simulink model "Dynamic_RLC_system"  (R2024a)
settings: Solver=VariableStepAuto  StartTime=0.0  StopTime=10.0  MaxStep=1e-3  RelTol=1e-3
settings Model: Creator=DELL  LastModifiedBy=DELL

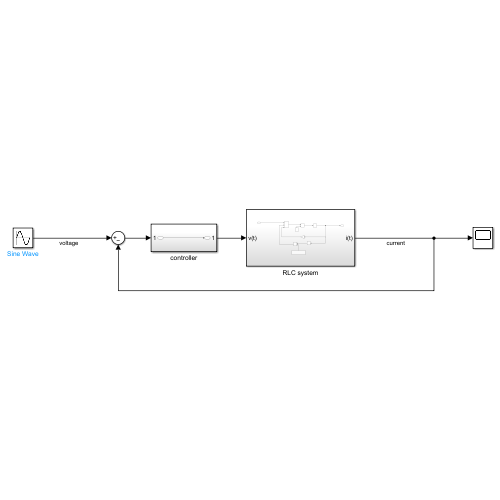
[thumbnail: Simulink's stored preview of the top-level diagram]
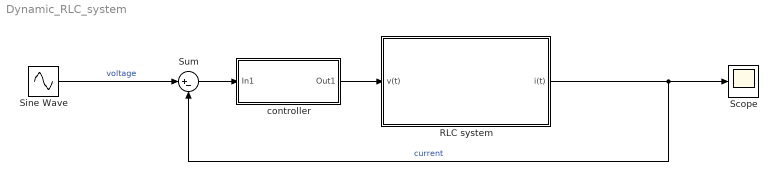
== system Dynamic_RLC_system ==
  RLC system : Subsystem
  Scope : Scope
  Sine Wave : Sin  Frequency=2000  SampleTime=0
  Sum : Sum  Inputs=|+-
  controller : Subsystem
  wires:
  RLC system/1(i(t)) -> Sum/2, Scope/1  "current"
  controller/1(Out1) -> RLC system/1(v(t))
  Sine Wave/1 -> Sum/1  "voltage"
  Sum/1 -> controller/1(In1)

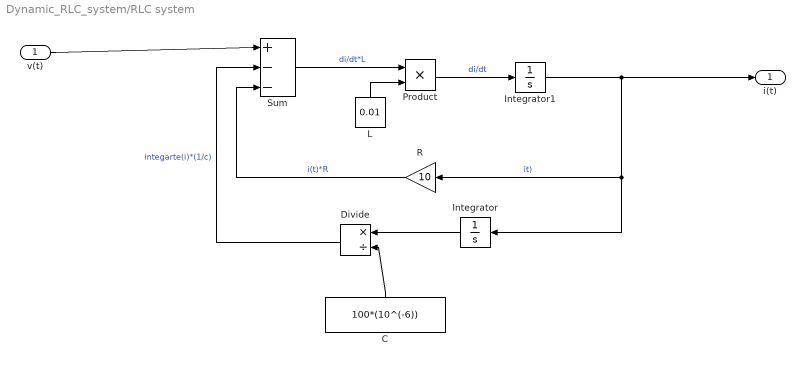
== system Dynamic_RLC_system/RLC system ==
  v(t) : Inport
  C : Constant  Value=100*(10^(-6))
  Divide : Product  Inputs=*/
  Integrator : Integrator
  Integrator1 : Integrator
  L : Constant  Value=0.01
  Product : Product
  R : Gain  Gain=10
  Sum : Sum  Inputs=|+|-|-
  i(t) : Outport
  wires:
  C/1 -> Divide/2
  L/1 -> Product/2
  Integrator1/1 -> i(t)/1, R/1, Integrator/1  "it)"
  Divide/1 -> Sum/2  "integarte(i)*(1/c)"
  Integrator/1 -> Divide/1
  Product/1 -> Integrator1/1  "di/dt"
  Sum/1 -> Product/1  "di/dt*L"
  R/1 -> Sum/3  "i(t)*R"
  v(t)/1 -> Sum/1

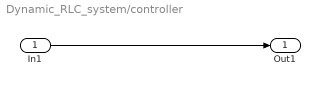
== system Dynamic_RLC_system/controller ==
  In1 : Inport
  Out1 : Outport
  wires:
  In1/1 -> Out1/1
